simulink model "TITO_OC_TC_2018"  (Simulink 9.1)
settings: Solver=ode45  StartTime=0.0  StopTime=100  RelTol=1e-3  EnableMultiTasking=on
libraries: simulink x3
settings Model: Creator=petr  LastModifiedBy=NICHOLAS ANG
settings DataIOCC: LimitDataPoints=on  SignalLoggingSaveFormat=ModelDataLogs
settings OptimizationCC: ExpressionDepthLimit=2147483647  InitFltsAndDblsToZero=on
settings DebuggingCC: SolverPrmCheckMsg=warning  FcnCallInpInsideContextMsg=warning  StateNameClashWarn=warning

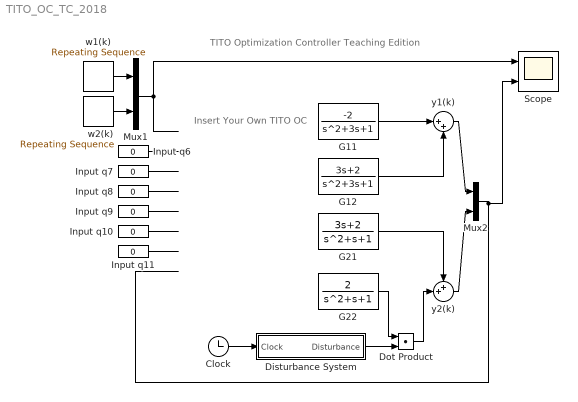
== system TITO_OC_TC_2018 ==
  note: TITO Optimization Controller Teaching Edition
  note: Insert Your Own
      | TITO OC
  Clock : Clock
  Disturbance System : Subsystem
  Dot Product : DotProduct  InputSameDT=on  OutDataTypeStr=Inherit: Inherit via internal rule
  G11 : TransferFcn  Numerator=[-2]  Denominator=[1 3 1]
  G12 : TransferFcn  Numerator=[3 2]  Denominator=[1 3 1]
  G21 : TransferFcn  Numerator=[3 2]  Denominator=[1 1 1]
  G22 : TransferFcn  Numerator=[2]  Denominator=[1 1 1]
  Input q{6..11} (6 alike) : Constant  Value=0
  Mux1 : Mux  Inputs=2
  Mux2 : Mux  Inputs=2
  "Scope  " : Scope  NumInputPorts=2
  w1(k) : simulink/Sources/Repeating Sequence  rep_seq_t=20*[0 0.4999 0.5 1.4999]  rep_seq_y=[1 1 2 2]
  w2(k) : simulink/Sources/Repeating Sequence  rep_seq_t=20*[0 0.9999 1.0 1.4999]  rep_seq_y=0.52*[1 1 2 2]
  y1(k) : Sum  Inputs=|++
  y2(k) : Sum  Inputs=++|
  wires:
  G12/1 -> y1(k)/2
  G21/1 -> y2(k)/1
  y2(k)/1 -> Mux2/2
  Input q6/1 -> ?
  Input q7/1 -> ?
  Input q8/1 -> ?
  Input q9/1 -> ?
  Input q10/1 -> ?
  Input q11/1 -> ?
  Mux2/1 -> "Scope  "/2
  w2(k)/1 -> Mux1/2
  Mux1/1 -> "Scope  "/1
  y1(k)/1 -> Mux2/1
  G11/1 -> y1(k)/1
  Disturbance System/1(Disturbance) -> Dot Product/2
  G22/1 -> Dot Product/1
  Dot Product/1 -> y2(k)/2
  Clock/1 -> Disturbance System/1(Clock)
  w1(k)/1 -> Mux1/1

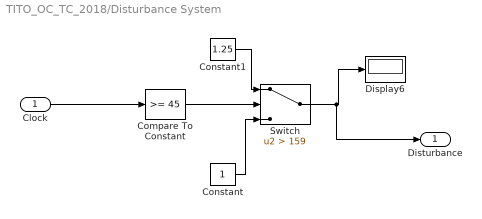
== system TITO_OC_TC_2018/Disturbance System ==
  Clock : Inport
  Compare To Constant : simulink/Logic and Bit Operations/Compare To Constant  relop=>=  const=45  OutDataTypeStr=boolean
  Constant : Constant
  Constant1 : Constant  Value=1.25
  Display6 : Display
  Switch : Switch  Criteria=u2 > Threshold  Threshold=159
  Disturbance : Outport
  wires:
  Compare To Constant/1 -> Switch/2
  Constant/1 -> Switch/3
  Constant1/1 -> Switch/1
  Switch/1 -> Disturbance/1, Display6/1
  Clock/1 -> Compare To Constant/1
